simulink library "WDB_Creator"  (R2013b)
settings: Solver=ode45  StartTime=0.0  StopTime=10.0  RelTol=1e-3
settings Model: Creator=drhf  LastModifiedBy=drhf

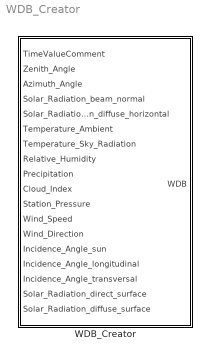
== system WDB_Creator ==
  WDB_Creator : Subsystem  mask(Weather Data Bus Creator){}
      mask help: Create the weather data bus with scalar inputs.
      mask Help: web(fullfile(path_carnot('help'),'WDB_Creator.html'),'-helpbrowser')

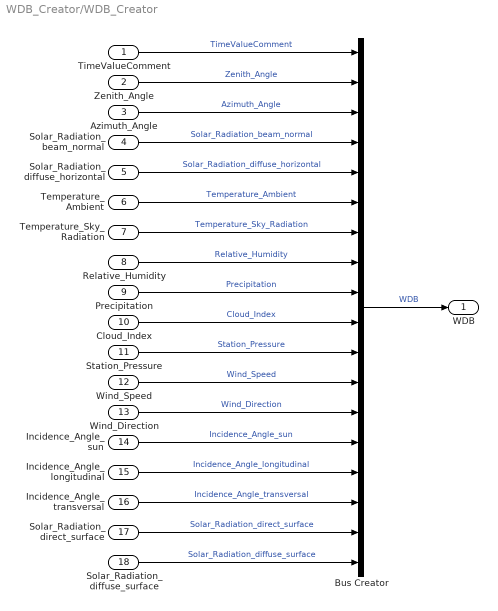
== system WDB_Creator/WDB_Creator ==
  TimeValueComment : Inport
  Zenith_Angle : Inport  Port=2
  Azimuth_Angle : Inport  Port=3
  Solar_Radiation_beam_normal : Inport  Port=4
  Solar_Radiation_diffuse_horizontal : Inport  Port=5
  Temperature_Ambient : Inport  Port=6
  Temperature_Sky_Radiation : Inport  Port=7
  Relative_Humidity : Inport  Port=8
  Precipitation : Inport  Port=9
  Cloud_Index : Inport  Port=10
  Station_Pressure : Inport  Port=11
  Wind_Speed : Inport  Port=12
  Wind_Direction : Inport  Port=13
  Incidence_Angle_sun : Inport  Port=14
  Incidence_Angle_longitudinal : Inport  Port=15
  Incidence_Angle_transversal : Inport  Port=16
  Solar_Radiation_direct_surface : Inport  Port=17
  Solar_Radiation_diffuse_surface : Inport  Port=18
  Bus Creator : BusCreator  InitFcn=load WDB.mat  Inputs=18  OutDataTypeStr=Bus: WDB
  WDB : Outport
  wires:
  Solar_Radiation_beam_normal/1 -> Bus Creator/4  "Solar_Radiation_beam_normal"
  TimeValueComment/1 -> Bus Creator/1  "TimeValueComment"
  Zenith_Angle/1 -> Bus Creator/2  "Zenith_Angle"
  Azimuth_Angle/1 -> Bus Creator/3  "Azimuth_Angle"
  Solar_Radiation_diffuse_horizontal/1 -> Bus Creator/5  "Solar_Radiation_diffuse_horizontal"
  Temperature_Ambient/1 -> Bus Creator/6  "Temperature_Ambient"
  Temperature_Sky_Radiation/1 -> Bus Creator/7  "Temperature_Sky_Radiation"
  Relative_Humidity/1 -> Bus Creator/8  "Relative_Humidity"
  Precipitation/1 -> Bus Creator/9  "Precipitation"
  Cloud_Index/1 -> Bus Creator/10  "Cloud_Index"
  Station_Pressure/1 -> Bus Creator/11  "Station_Pressure"
  Wind_Speed/1 -> Bus Creator/12  "Wind_Speed"
  Wind_Direction/1 -> Bus Creator/13  "Wind_Direction"
  Incidence_Angle_sun/1 -> Bus Creator/14  "Incidence_Angle_sun"
  Incidence_Angle_longitudinal/1 -> Bus Creator/15  "Incidence_Angle_longitudinal"
  Incidence_Angle_transversal/1 -> Bus Creator/16  "Incidence_Angle_transversal"
  Solar_Radiation_direct_surface/1 -> Bus Creator/17  "Solar_Radiation_direct_surface"
  Solar_Radiation_diffuse_surface/1 -> Bus Creator/18  "Solar_Radiation_diffuse_surface"
  Bus Creator/1 -> WDB/1  "WDB"
